simulink model "lab2_model_ssEmulation_choices"  (R2024b)
settings: Solver=VariableStepAuto  StartTime=0.0  StopTime=sIn.simulation_time  FixedStep=sIn.step_size  MaxStep=sIn.step_size
undefined symbols (not defined in the file or in its folder): DiscIntNeverNeededParam, feedback, obs, rpm2rads, sens, sIn
settings Model: Creator=bmm1  LastModifiedBy=pries
settings DataIOCC: ReturnWorkspaceOutputs=off
settings RTWCC: GPUComputeCapability=3.5

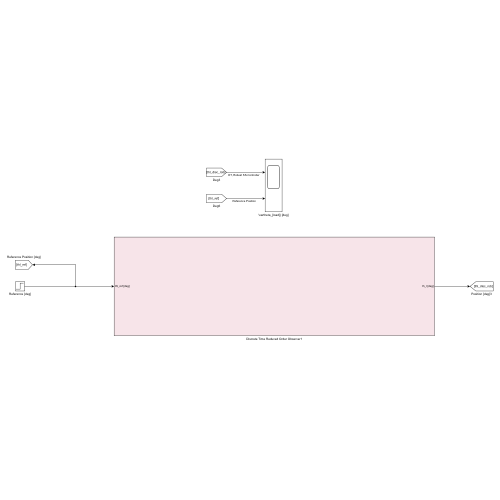
[thumbnail: Simulink's stored preview of the top-level diagram]
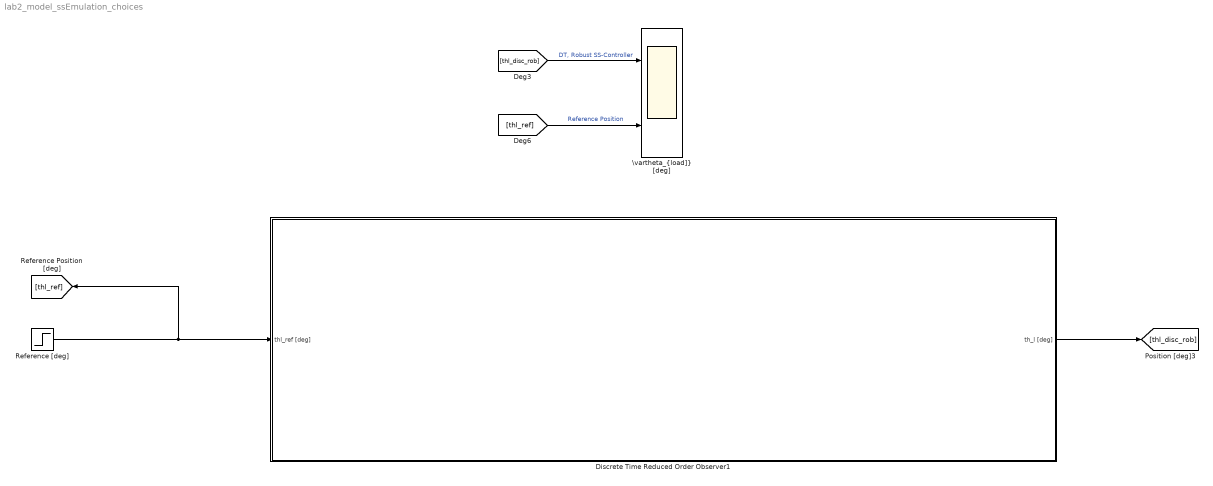
== system lab2_model_ssEmulation_choices ==
  Discrete Time Reduced Order Observer1 : Subsystem
  Reference [deg] : Step  Time=0  After=sIn.position  SampleTime=0
  "\\vartheta_{load]} [deg]" : Scope  NumInputPorts=2
  wires:
  [thl_ref] -> "\\vartheta_{load]} [deg]"/2  "Reference Position"
  Reference [deg]/1 -> Discrete Time Reduced Order Observer1/1(thl_ref [deg]), [thl_ref]
  Discrete Time Reduced Order Observer1/1(th_l [deg]) -> [thl_disc_rob]
  [thl_disc_rob] -> "\\vartheta_{load]} [deg]"/1  "DT, Robust SS-Controller"

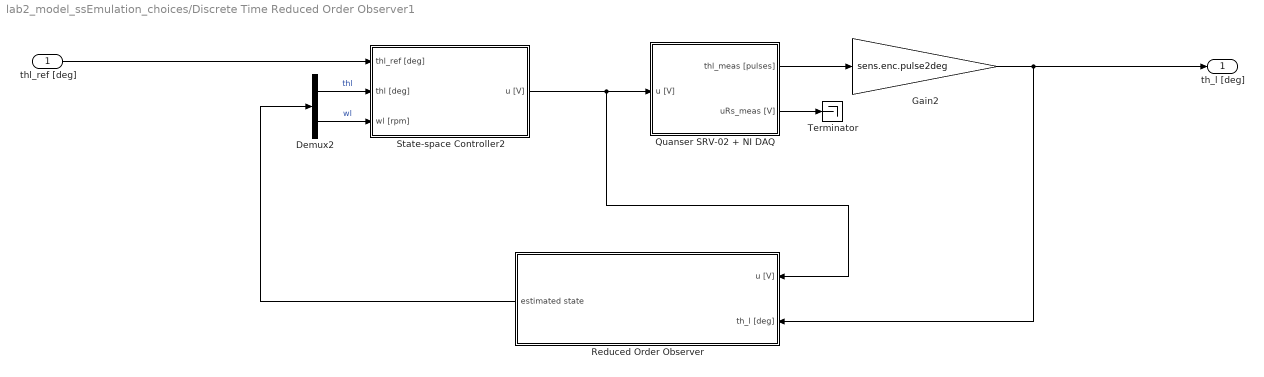
== system lab2_model_ssEmulation_choices/Discrete Time Reduced Order Observer1 ==
  thl_ref [deg] : Inport
  Demux2 : Demux  Outputs=2
  Gain2 : Gain  Gain=sens.enc.pulse2deg
  Quanser SRV-02 + NI DAQ : Subsystem  mask(Quanser SRV-02 (with inertial load) + NI DAQ){Ts=0.001, fricType=Coulomb + viscous}
      mask prompts: Ts "NI DAQ Sample Time:"; fricType "Friction model"
      mask help: Quanser SRV-02 (with inertial load) + NI DAQ model.
      mask init:
      | %%  Sensors data
      | 
      | %   shunt resistor
      | sens.curr.Rs = 0.5;                         %   resistance [Ohm]   
      | sens.curr.uRs_std = 0.01;                   %   voltage noise standard dev [V]                           
      | sens.curr.uRs_var = sens.curr.uRs_std^2;	%   voltage noise variance [V^2]
      | 
      | %   Hewlett-Packard HEDS-5540#A06 optical encoder
      | sens.enc.ppr = 500*4;                       %   pulses per rotation
      | sens.enc.pulse2deg = 360/sens.enc.ppr;      %   [pulses] -> [deg]
      | sens.enc.pulse2rad = 2*pi/sens.enc.ppr;     %   [pulses] -> [rad]
      | sens.enc.deg2pulse = sens.enc.ppr/360;      %   [deg] -> [pulses]
      | sens.enc.rad2pulse = sens.enc.ppr/2/pi;     %   [rad] -> [pulses]
      | 
      | 
      | %%  Data acquisition board (daq) data
      | 
      | %   NI PCI-6221 DAC data
      | daq.dac.bits = 16;                                  %   resolution (bits)
      | daq.dac.fs   = 10;                                  %   full scale 
      | daq.dac.q    = 2*daq.dac.fs/(2^daq.dac.bits-1);     %	quantization
      | 
      | %   NI PCI-6221 ADC data
      | daq.adc.bits = 16;                                  %   resolution (bits)
      | daq.adc.fs   = 10;                                  %   full scale (as set in SLDRT Analog Input block)
      | daq.adc.q    = 2*daq.adc.fs/(2^daq.adc.bits-1);     %   quantization
      mask Help:
      | Riccardo Antonello (antonello@dei.unipd.it)
      | 
      | April 24, 2020
      | 
      | Dept. of Information Engineering, University of Padova
      mask TypeOptions fricType: Coulomb + viscous | Karnopp
  Reduced Order Observer : Subsystem
  State-space Controller2 : Subsystem
  Terminator : Terminator
  th_l [deg] : Outport
  wires:
  thl_ref [deg]/1 -> State-space Controller2/1(thl_ref [deg])
  Demux2/1 -> State-space Controller2/2(thl [deg])  "thl"
  Demux2/2 -> State-space Controller2/3(wl [rpm])  "wl"
  Quanser SRV-02 + NI DAQ/1(thl_meas [pulses]) -> Gain2/1
  Gain2/1 -> Reduced Order Observer/2(th_l [deg]), th_l [deg]/1
  State-space Controller2/1(u [V]) -> Quanser SRV-02 + NI DAQ/1(u [V]), Reduced Order Observer/1(u [V])
  Reduced Order Observer/1(estimated state) -> Demux2/1
  Quanser SRV-02 + NI DAQ/2(uRs_meas [V]) -> Terminator/1

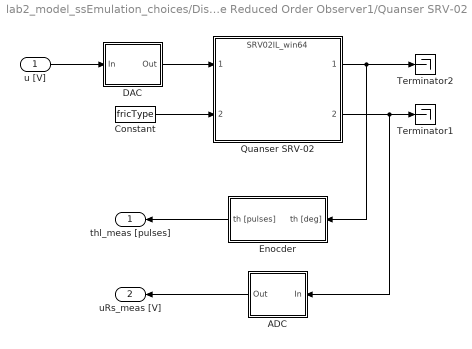
== system lab2_model_ssEmulation_choices/Discrete Time Reduced Order Observer1/Quanser SRV-02 + NI DAQ ==
  u [V] : Inport
  ADC : Subsystem
  Constant : Constant  Value=fricType
  DAC : Subsystem
  Enocder : Subsystem
  Quanser SRV-02 : ModelReference  ModelNameDialog=SRV02IL_win64.slxp  ModelReferenceVersion=1.44  CopyOfModelProtected=on
  Terminator1 : Terminator
  Terminator2 : Terminator
  thl_meas [pulses] : Outport
  uRs_meas [V] : Outport  Port=2
  wires:
  Enocder/1(th [pulses]) -> thl_meas [pulses]/1
  ADC/1(Out) -> uRs_meas [V]/1
  DAC/1(Out) -> Quanser SRV-02/1
  Quanser SRV-02/2 -> ADC/1(In), Terminator1/1
  u [V]/1 -> DAC/1(In)
  Quanser SRV-02/1 -> Enocder/1(th [deg]), Terminator2/1
  Constant/1 -> Quanser SRV-02/2

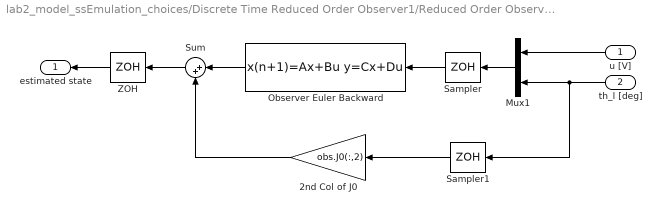
== system lab2_model_ssEmulation_choices/Discrete Time Reduced Order Observer1/Reduced Order Observer ==
  u [V] : Inport
  th_l [deg] : Inport  Port=2
  2nd Col of J0 : Gain  Gain=obs.J0(:,2)
  Mux1 : Mux  Inputs=2
  Observer Euler Backward : DiscreteStateSpace  A=obs.Phi0  B=obs.Gamma0  C=obs.H0  D=zeros(2,2)  SampleTime=sIn.T_s
  Sampler : ZeroOrderHold  SampleTime=sIn.T_s
  Sampler1 : ZeroOrderHold  SampleTime=sIn.T_s
  Sum : Sum  Inputs=|++
  ZOH : ZeroOrderHold  SampleTime=sIn.T_s
  estimated state : Outport
  wires:
  Sampler/1 -> Observer Euler Backward/1
  Sum/1 -> ZOH/1
  Observer Euler Backward/1 -> Sum/1
  Sampler1/1 -> 2nd Col of J0/1
  Mux1/1 -> Sampler/1
  2nd Col of J0/1 -> Sum/2
  th_l [deg]/1 -> Mux1/2, Sampler1/1
  u [V]/1 -> Mux1/1
  ZOH/1 -> estimated state/1

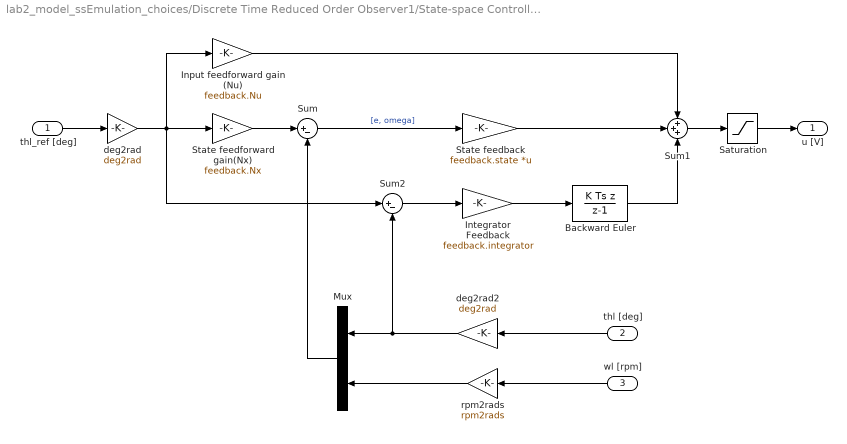
== system lab2_model_ssEmulation_choices/Discrete Time Reduced Order Observer1/State-space Controller2 ==
  thl_ref [deg] : Inport
  thl [deg] : Inport  Port=2
  wl [rpm] : Inport  Port=3
  Backward Euler : DiscreteIntegrator  IntegratorMethod=Integration: Backward Euler  SampleTime=sIn.T_s  ICPrevOutput=DiscIntNeverNeededParam  ICPrevScaledInput=DiscIntNeverNeededParam
  Input feedforward gain (Nu) : Gain  Gain=feedback.Nu
  Integrator Feedback : Gain  Gain=feedback.integrator
  Mux : Mux  Inputs=2
  Saturation : Saturate  UpperLimit=10  LowerLimit=-10
  State feedback : Gain  Gain=feedback.state  Multiplication=Matrix(K*u)
  State feedforward gain(Nx) : Gain  Gain=feedback.Nx
  Sum : Sum  Inputs=|+-
  Sum1 : Sum  Inputs=+++
  Sum2 : Sum  Inputs=|+-
  deg2rad : Gain  Gain=deg2rad
  deg2rad2 : Gain  Gain=deg2rad
  rpm2rads : Gain  Gain=rpm2rads
  u [V] : Outport
  wires:
  thl_ref [deg]/1 -> deg2rad/1
  deg2rad/1 -> State feedforward gain(Nx)/1, Input feedforward gain (Nu)/1, Sum2/1
  State feedforward gain(Nx)/1 -> Sum/1
  Sum/1 -> State feedback/1  "[e, omega]"
  Sum1/1 -> Saturation/1
  Saturation/1 -> u [V]/1
  thl [deg]/1 -> deg2rad2/1
  wl [rpm]/1 -> rpm2rads/1
  deg2rad2/1 -> Sum2/2, Mux/1
  rpm2rads/1 -> Mux/2
  Mux/1 -> Sum/2
  Sum2/1 -> Integrator Feedback/1
  Backward Euler/1 -> Sum1/3
  Input feedforward gain (Nu)/1 -> Sum1/1
  State feedback/1 -> Sum1/2
  Integrator Feedback/1 -> Backward Euler/1

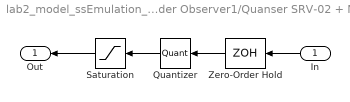
== system lab2_model_ssEmulation_choices/Discrete Time Reduced Order Observer1/Quanser SRV-02 + NI DAQ/ADC ==
  In : Inport
  Quantizer : Quantizer  QuantizationInterval=daq.adc.q
  Saturation : Saturate  UpperLimit=daq.adc.fs  LowerLimit=-daq.adc.fs
  Zero-Order Hold : ZeroOrderHold  SampleTime=Ts
  Out : Outport
  wires:
  Saturation/1 -> Out/1
  In/1 -> Zero-Order Hold/1
  Quantizer/1 -> Saturation/1
  Zero-Order Hold/1 -> Quantizer/1

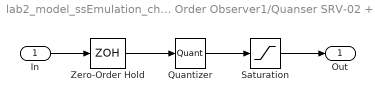
== system lab2_model_ssEmulation_choices/Discrete Time Reduced Order Observer1/Quanser SRV-02 + NI DAQ/DAC ==
  In : Inport
  Quantizer : Quantizer  QuantizationInterval=daq.dac.q
  Saturation : Saturate  UpperLimit=daq.dac.fs  LowerLimit=-daq.dac.fs
  Zero-Order Hold : ZeroOrderHold  SampleTime=Ts
  Out : Outport
  wires:
  Quantizer/1 -> Saturation/1
  In/1 -> Zero-Order Hold/1
  Zero-Order Hold/1 -> Quantizer/1
  Saturation/1 -> Out/1

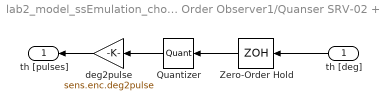
== system lab2_model_ssEmulation_choices/Discrete Time Reduced Order Observer1/Quanser SRV-02 + NI DAQ/Enocder ==
  th [deg] : Inport
  Quantizer : Quantizer  QuantizationInterval=sens.enc.pulse2deg
  Zero-Order Hold : ZeroOrderHold  SampleTime=Ts
  deg2pulse : Gain  Gain=sens.enc.deg2pulse
  th [pulses] : Outport
  wires:
  Quantizer/1 -> deg2pulse/1
  th [deg]/1 -> Zero-Order Hold/1
  Zero-Order Hold/1 -> Quantizer/1
  deg2pulse/1 -> th [pulses]/1
